simulink model "model"  (R2020a)
settings: Solver=VariableStepAuto  StartTime=0.0  StopTime=10.0  RelTol=1e-3
settings Model: Creator=PRATIKSHA  LastModifiedBy=PRATIKSHA

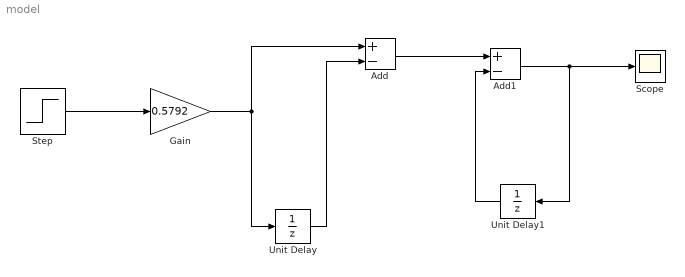
== system model ==
  Add : Sum  Inputs=+-
  Add1 : Sum  Inputs=+-
  Gain : Gain  Gain=0.5792
  Scope : Scope
  Step : Step  SampleTime=0
  Unit Delay : UnitDelay  SampleTime=-1  HasFrameUpgradeWarning=on
  Unit Delay1 : UnitDelay  SampleTime=-1  HasFrameUpgradeWarning=on
  wires:
  Step/1 -> Gain/1
  Add/1 -> Add1/1
  Unit Delay1/1 -> Add1/2
  Gain/1 -> Unit Delay/1, Add/1
  Unit Delay/1 -> Add/2
  Add1/1 -> Scope/1, Unit Delay1/1
